simulink model "babybox"  (R2018a)
settings: Solver=VariableStepAuto  StartTime=0.0  StopTime=10.0  RelTol=1e-3
settings Model: Creator=BEAR  LastModifiedBy=BEAR

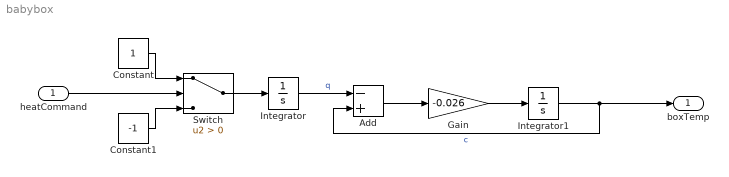
== system babybox ==
  heatCommand : Inport
  Add : Sum  Inputs=-+
  Constant : Constant
  Constant1 : Constant  Value=-1
  Gain : Gain  Gain=-0.026
  Integrator : Integrator  InitialCondition=97
  Integrator1 : Integrator  InitialCondition=100
  Switch : Switch  Criteria=u2 > Threshold
  boxTemp : Outport
  wires:
  Constant/1 -> Switch/1
  Switch/1 -> Integrator/1
  Integrator/1 -> Add/1  "q"
  Add/1 -> Gain/1
  Gain/1 -> Integrator1/1
  heatCommand/1 -> Switch/2
  Constant1/1 -> Switch/3
  Integrator1/1 -> Add/2, boxTemp/1  "c"
